simulink model "system_back_end"  (R2023a)
settings: Solver=VariableStepAuto  StartTime=0.0  StopTime=10.0  RelTol=1e-3
settings Model: Creator=Cinovasi  LastModifiedBy=Cinovasi

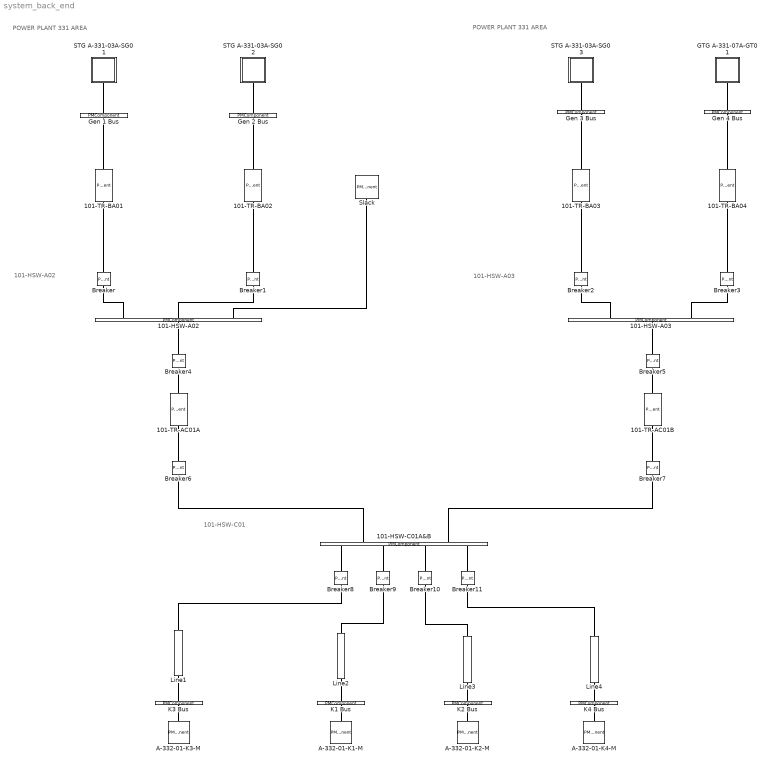
== system system_back_end ==
  note: 101-HSW-A03
  note: 101-HSW-A02
  note: 101-HSW-C01
  note: POWER PLANT 331 AREA
  note: POWER PLANT 331 AREA
  101-HSW-A02 : PMComponent  Tag=PSATblock  Description=Connection  PhysicalDomain=psatdomain  LeftPortType=p1  RightPortType=p1  LConnTagsString=__newl0|__newl1|__newl2  RConnTagsString=__newr0  mask(Bus){in=3, out=1, p2q=33, p3_4q=[1.00  0.00], p5q=1, p6q=1}
      mask prompts: in "Number of inputs:"; out "Number of outputs:"; p2q "Voltage Rating [kV]"; p3_4q "Voltage initial guess [p.u.  rad]"; p5q "Area number"; p6q "Region number"
      mask help: Bus block.
      mask init:
      | fm_inout
      mask Callback p5q: fm_block
      mask Display: plot([0 1 1 0 0],[0 0 1 1 0])
  101-HSW-A03 : PMComponent  Tag=PSATblock  Description=Connection  PhysicalDomain=psatdomain  LeftPortType=p1  RightPortType=p1  LConnTagsString=__newl0|__newl1  RConnTagsString=__newr0  mask(Bus){in=2, out=1, p2q=33, p3_4q=[1.00  0.00], p5q=1, p6q=1}
      mask prompts: in "Number of inputs:"; out "Number of outputs:"; p2q "Voltage Rating [kV]"; p3_4q "Voltage initial guess [p.u.  rad]"; p5q "Area number"; p6q "Region number"
      mask help: Bus block.
      mask init:
      | fm_inout
      mask Callback p5q: fm_block
      mask Display: plot([0 1 1 0 0],[0 0 1 1 0])
  101-HSW-C01A&B : PMComponent  Tag=PSATblock  Description=Connection  PhysicalDomain=psatdomain  LeftPortType=p1  RightPortType=p1  LConnTagsString=__newl0|__newl1  RConnTagsString=__newr0|__newr1|__newr2|__newr3  mask(Bus){in=2, out=4, p2q=5, p3_4q=[1.00  0.00], p5q=1, p6q=1}
      mask prompts: in "Number of inputs:"; out "Number of outputs:"; p2q "Voltage Rating [kV]"; p3_4q "Voltage initial guess [p.u.  rad]"; p5q "Area number"; p6q "Region number"
      mask help: Bus block.
      mask init:
      | fm_inout
      mask Callback p5q: fm_block
      mask Display: plot([0 1 1 0 0],[0 0 1 1 0])
  101-TR-AC01A : PMComponent  Tag=PSATblock  Description=Power Flow  PhysicalDomain=psatdomain  LeftPortType=p1  RightPortType=p1  LConnTagsString=__newl0  RConnTagsString=__newr0  mask(Line){p3_4_5q=[40 33 50], p7q=33/7, p8q=0.01, p9q=0.20, p13_14_15q=[0.0  0.0  0.0], p16q=on}
      mask prompts: p3_4_5q "Power, Voltage and Frequency Ratings [MVA, kV, Hz]"; p7q "Primary and secondary voltage ratio [kV/kV]"; p8q "Resistance [p.u.]"; p9q "Reactance [p.u.]"; p13_14_15q "Imax, Pmax and Smax [p.u., p.u., p.u.]"; p16q "Connected"
      mask help: This block defines a transformer.
      mask init:
      | [x,y] = fm_draw('circle');
      | [x1,y1] = fm_draw('1');
      | [x2,y2] = fm_draw('2');
      mask Callback p16q: fm_block
      mask Display:
      | plot(x,y,x+1.4,y,[-1 -1.3],[0 0],[2.4 2.7],[0 0])
      | color('green')
      | plot(-0.1+0.65*x1,0.65*y1)
      | plot(1.5+0.65*x2,0.65*y2)
  101-TR-AC01B : PMComponent  Tag=PSATblock  Description=Power Flow  PhysicalDomain=psatdomain  LeftPortType=p1  RightPortType=p1  LConnTagsString=__newl0  RConnTagsString=__newr0  mask(Line){p3_4_5q=[40 33 50], p7q=33/7, p8q=0.01, p9q=0.20, p13_14_15q=[0.0  0.0  0.0], p16q=on}
      mask prompts: p3_4_5q "Power, Voltage and Frequency Ratings [MVA, kV, Hz]"; p7q "Primary and secondary voltage ratio [kV/kV]"; p8q "Resistance [p.u.]"; p9q "Reactance [p.u.]"; p13_14_15q "Imax, Pmax and Smax [p.u., p.u., p.u.]"; p16q "Connected"
      mask help: This block defines a transformer.
      mask init:
      | [x,y] = fm_draw('circle');
      | [x1,y1] = fm_draw('1');
      | [x2,y2] = fm_draw('2');
      mask Callback p16q: fm_block
      mask Display:
      | plot(x,y,x+1.4,y,[-1 -1.3],[0 0],[2.4 2.7],[0 0])
      | color('green')
      | plot(-0.1+0.65*x1,0.65*y1)
      | plot(1.5+0.65*x2,0.65*y2)
  101-TR-BA01 : PMComponent  Tag=PSATblock  Description=Power Flow  PhysicalDomain=psatdomain  LeftPortType=p1  RightPortType=p1  LConnTagsString=__newl0  RConnTagsString=__newr0  mask(Line){p3_4_5q=[40 11 50], p7q=11/20, p8q=0.01, p9q=0.20, p13_14_15q=[0.0  0.0  0.0], p16q=on}
      mask prompts: p3_4_5q "Power, Voltage and Frequency Ratings [MVA, kV, Hz]"; p7q "Primary and secondary voltage ratio [kV/kV]"; p8q "Resistance [p.u.]"; p9q "Reactance [p.u.]"; p13_14_15q "Imax, Pmax and Smax [p.u., p.u., p.u.]"; p16q "Connected"
      mask help: This block defines a transformer.
      mask init:
      | [x,y] = fm_draw('circle');
      | [x1,y1] = fm_draw('1');
      | [x2,y2] = fm_draw('2');
      mask Callback p16q: fm_block
      mask Display:
      | plot(x,y,x+1.4,y,[-1 -1.3],[0 0],[2.4 2.7],[0 0])
      | color('green')
      | plot(-0.1+0.65*x1,0.65*y1)
      | plot(1.5+0.65*x2,0.65*y2)
  101-TR-BA02 : PMComponent  Tag=PSATblock  Description=Power Flow  PhysicalDomain=psatdomain  LeftPortType=p1  RightPortType=p1  LConnTagsString=__newl0  RConnTagsString=__newr0  mask(Line){p3_4_5q=[40 11 50], p7q=11/20, p8q=0.01, p9q=0.20, p13_14_15q=[0.0  0.0  0.0], p16q=on}
      mask prompts: p3_4_5q "Power, Voltage and Frequency Ratings [MVA, kV, Hz]"; p7q "Primary and secondary voltage ratio [kV/kV]"; p8q "Resistance [p.u.]"; p9q "Reactance [p.u.]"; p13_14_15q "Imax, Pmax and Smax [p.u., p.u., p.u.]"; p16q "Connected"
      mask help: This block defines a transformer.
      mask init:
      | [x,y] = fm_draw('circle');
      | [x1,y1] = fm_draw('1');
      | [x2,y2] = fm_draw('2');
      mask Callback p16q: fm_block
      mask Display:
      | plot(x,y,x+1.4,y,[-1 -1.3],[0 0],[2.4 2.7],[0 0])
      | color('green')
      | plot(-0.1+0.65*x1,0.65*y1)
      | plot(1.5+0.65*x2,0.65*y2)
  101-TR-BA03 : PMComponent  Tag=PSATblock  Description=Power Flow  PhysicalDomain=psatdomain  LeftPortType=p1  RightPortType=p1  LConnTagsString=__newl0  RConnTagsString=__newr0  mask(Line){p3_4_5q=[40 11 50], p7q=11/20, p8q=0.01, p9q=0.20, p13_14_15q=[0.0  0.0  0.0], p16q=on}
      mask prompts: p3_4_5q "Power, Voltage and Frequency Ratings [MVA, kV, Hz]"; p7q "Primary and secondary voltage ratio [kV/kV]"; p8q "Resistance [p.u.]"; p9q "Reactance [p.u.]"; p13_14_15q "Imax, Pmax and Smax [p.u., p.u., p.u.]"; p16q "Connected"
      mask help: This block defines a transformer.
      mask init:
      | [x,y] = fm_draw('circle');
      | [x1,y1] = fm_draw('1');
      | [x2,y2] = fm_draw('2');
      mask Callback p16q: fm_block
      mask Display:
      | plot(x,y,x+1.4,y,[-1 -1.3],[0 0],[2.4 2.7],[0 0])
      | color('green')
      | plot(-0.1+0.65*x1,0.65*y1)
      | plot(1.5+0.65*x2,0.65*y2)
  101-TR-BA04 : PMComponent  Tag=PSATblock  Description=Power Flow  PhysicalDomain=psatdomain  LeftPortType=p1  RightPortType=p1  LConnTagsString=__newl0  RConnTagsString=__newr0  mask(Line){p3_4_5q=[40 11 50], p7q=11/20, p8q=0.01, p9q=0.20, p13_14_15q=[0.0  0.0  0.0], p16q=on}
      mask prompts: p3_4_5q "Power, Voltage and Frequency Ratings [MVA, kV, Hz]"; p7q "Primary and secondary voltage ratio [kV/kV]"; p8q "Resistance [p.u.]"; p9q "Reactance [p.u.]"; p13_14_15q "Imax, Pmax and Smax [p.u., p.u., p.u.]"; p16q "Connected"
      mask help: This block defines a transformer.
      mask init:
      | [x,y] = fm_draw('circle');
      | [x1,y1] = fm_draw('1');
      | [x2,y2] = fm_draw('2');
      mask Callback p16q: fm_block
      mask Display:
      | plot(x,y,x+1.4,y,[-1 -1.3],[0 0],[2.4 2.7],[0 0])
      | color('green')
      | plot(-0.1+0.65*x1,0.65*y1)
      | plot(1.5+0.65*x2,0.65*y2)
  A-332-01-K1-M : PMComponent  Tag=PSATblock  Description=Machines  PhysicalDomain=psatdomain  LeftPortType=p1  RightPortType=p1  LConnTagsString=__newl0  mask(Ind){p2_3_4q=[40 6.6 50], p5q=3, p6q=off, p7q=0.01, p8q=0.15, p9_10q=[0.05  0.15], p11_12q=[0.001  0.04], p13q=5.00, p14q=3.00, p15_16_17q=[1.00  0.00  0.00], p18q=0, p19q=off, p20q=on}
      mask prompts: p2_3_4q "Power, Voltage and Frequency Ratings [MVA, kV, Hz]"; p5q "Dynamic Order"; p6q "Start up"; p7q "Stator Resistance Rs [p.u.]"; p8q "Stator Reactance Xs [p.u.]"; p9_10q "First Cage Resitance Rr1 and Reactance  Xr1 [p.u. p.u.]"; p11_12q "Second Cage Resistance Rr2 and Reactance Xr2 [p.u.  p.u.]"; p13q "Magnetization Reactance Xm [p.u.]"; p14q "Inertia Constant Hm [kWs/kVA]"; p15_16_17q "Mechanical Torque coefficients [a, b, c] [p.u.  p.u.  p.u.]"; p18q "Start up time"; p19q "Allow working as brake"; p20q "Connected"
      mask help:
      | This block defines an asynchronous machine.
      |
      | Order 1:  mechanical equation
      | Order 3:  single cage
      | Order 5:  double cage
      mask init:
      | [x,y] = fm_draw('circle');
      | [xs,ys] = fm_draw('sinus');
      mask TypeOptions p5q: 1 | 3 | 5
      mask Callback p5q: fm_block
      mask Callback p20q: fm_block
      mask Display:
      | plot(x+1.4,y,0.12*xs+1,0.15*ys-0.6)
      | color('blue')
      | plot([1 1 1.4 1.8 1.8],[-0.05 0.7 0.4 0.7 -0.05])
  A-332-01-K2-M : PMComponent  Tag=PSATblock  Description=Machines  PhysicalDomain=psatdomain  LeftPortType=p1  RightPortType=p1  LConnTagsString=__newl0  mask(Ind){p2_3_4q=[40 6.6 50], p5q=3, p6q=off, p7q=0.01, p8q=0.15, p9_10q=[0.05  0.15], p11_12q=[0.001  0.04], p13q=5.00, p14q=3.00, p15_16_17q=[1.00  0.00  0.00], p18q=0, p19q=off, p20q=on}
      mask prompts: p2_3_4q "Power, Voltage and Frequency Ratings [MVA, kV, Hz]"; p5q "Dynamic Order"; p6q "Start up"; p7q "Stator Resistance Rs [p.u.]"; p8q "Stator Reactance Xs [p.u.]"; p9_10q "First Cage Resitance Rr1 and Reactance  Xr1 [p.u. p.u.]"; p11_12q "Second Cage Resistance Rr2 and Reactance Xr2 [p.u.  p.u.]"; p13q "Magnetization Reactance Xm [p.u.]"; p14q "Inertia Constant Hm [kWs/kVA]"; p15_16_17q "Mechanical Torque coefficients [a, b, c] [p.u.  p.u.  p.u.]"; p18q "Start up time"; p19q "Allow working as brake"; p20q "Connected"
      mask help:
      | This block defines an asynchronous machine.
      |
      | Order 1:  mechanical equation
      | Order 3:  single cage
      | Order 5:  double cage
      mask init:
      | [x,y] = fm_draw('circle');
      | [xs,ys] = fm_draw('sinus');
      mask TypeOptions p5q: 1 | 3 | 5
      mask Callback p5q: fm_block
      mask Callback p20q: fm_block
      mask Display:
      | plot(x+1.4,y,0.12*xs+1,0.15*ys-0.6)
      | color('blue')
      | plot([1 1 1.4 1.8 1.8],[-0.05 0.7 0.4 0.7 -0.05])
  A-332-01-K3-M : PMComponent  Tag=PSATblock  Description=Machines  PhysicalDomain=psatdomain  LeftPortType=p1  RightPortType=p1  LConnTagsString=__newl0  mask(Ind){p2_3_4q=[40 6.6 50], p5q=3, p6q=off, p7q=0.01, p8q=0.15, p9_10q=[0.05  0.15], p11_12q=[0.001  0.04], p13q=5.00, p14q=3.00, p15_16_17q=[1.00  0.00  0.00], p18q=0, p19q=off, p20q=on}
      mask prompts: p2_3_4q "Power, Voltage and Frequency Ratings [MVA, kV, Hz]"; p5q "Dynamic Order"; p6q "Start up"; p7q "Stator Resistance Rs [p.u.]"; p8q "Stator Reactance Xs [p.u.]"; p9_10q "First Cage Resitance Rr1 and Reactance  Xr1 [p.u. p.u.]"; p11_12q "Second Cage Resistance Rr2 and Reactance Xr2 [p.u.  p.u.]"; p13q "Magnetization Reactance Xm [p.u.]"; p14q "Inertia Constant Hm [kWs/kVA]"; p15_16_17q "Mechanical Torque coefficients [a, b, c] [p.u.  p.u.  p.u.]"; p18q "Start up time"; p19q "Allow working as brake"; p20q "Connected"
      mask help:
      | This block defines an asynchronous machine.
      |
      | Order 1:  mechanical equation
      | Order 3:  single cage
      | Order 5:  double cage
      mask init:
      | [x,y] = fm_draw('circle');
      | [xs,ys] = fm_draw('sinus');
      mask TypeOptions p5q: 1 | 3 | 5
      mask Callback p5q: fm_block
      mask Callback p20q: fm_block
      mask Display:
      | plot(x+1.4,y,0.12*xs+1,0.15*ys-0.6)
      | color('blue')
      | plot([1 1 1.4 1.8 1.8],[-0.05 0.7 0.4 0.7 -0.05])
  A-332-01-K4-M : PMComponent  Tag=PSATblock  Description=Machines  PhysicalDomain=psatdomain  LeftPortType=p1  RightPortType=p1  LConnTagsString=__newl0  mask(Ind){p2_3_4q=[40 6.6 50], p5q=3, p6q=off, p7q=0.01, p8q=0.15, p9_10q=[0.05  0.15], p11_12q=[0.001  0.04], p13q=5.00, p14q=3.00, p15_16_17q=[1.00  0.00  0.00], p18q=0, p19q=off, p20q=on}
      mask prompts: p2_3_4q "Power, Voltage and Frequency Ratings [MVA, kV, Hz]"; p5q "Dynamic Order"; p6q "Start up"; p7q "Stator Resistance Rs [p.u.]"; p8q "Stator Reactance Xs [p.u.]"; p9_10q "First Cage Resitance Rr1 and Reactance  Xr1 [p.u. p.u.]"; p11_12q "Second Cage Resistance Rr2 and Reactance Xr2 [p.u.  p.u.]"; p13q "Magnetization Reactance Xm [p.u.]"; p14q "Inertia Constant Hm [kWs/kVA]"; p15_16_17q "Mechanical Torque coefficients [a, b, c] [p.u.  p.u.  p.u.]"; p18q "Start up time"; p19q "Allow working as brake"; p20q "Connected"
      mask help:
      | This block defines an asynchronous machine.
      |
      | Order 1:  mechanical equation
      | Order 3:  single cage
      | Order 5:  double cage
      mask init:
      | [x,y] = fm_draw('circle');
      | [xs,ys] = fm_draw('sinus');
      mask TypeOptions p5q: 1 | 3 | 5
      mask Callback p5q: fm_block
      mask Callback p20q: fm_block
      mask Display:
      | plot(x+1.4,y,0.12*xs+1,0.15*ys-0.6)
      | color('blue')
      | plot([1 1 1.4 1.8 1.8],[-0.05 0.7 0.4 0.7 -0.05])
  Breaker : PMComponent  Tag=PSATblock  Description=Faults & Breakers  PhysicalDomain=psatdomain  LeftPortType=p1  RightPortType=p1  LConnTagsString=__newl0  RConnTagsString=__newr0  mask(Breaker){p3_4_5q=[40 34.5  50], p6q=on, p7q=0.00, p8q=0.00, p9q=on, p10q=on}
      mask prompts: p3_4_5q "Power, Voltage and Frequency Ratings [MVA, kV, Hz]"; p6q "Initially close"; p7q "First intervention time [s]"; p8q "Second intervention time [s]"; p9q "Apply first intervention"; p10q "Apply second intervention"
      mask help: This block defines a transmission line breaker.
      mask Callback p6q: fm_block
      mask Display: plot([1 2 2 1 1],[-1 -1 1 1 -1]),color('red'),plot([1 2],[-1 1],[2 1],[-1 1])
  Breaker1 : PMComponent  Tag=PSATblock  Description=Faults & Breakers  PhysicalDomain=psatdomain  LeftPortType=p1  RightPortType=p1  LConnTagsString=__newl0  RConnTagsString=__newr0  mask(Breaker){p3_4_5q=[40 34.5  50], p6q=on, p7q=0.00, p8q=0.00, p9q=on, p10q=on}
      mask prompts: p3_4_5q "Power, Voltage and Frequency Ratings [MVA, kV, Hz]"; p6q "Initially close"; p7q "First intervention time [s]"; p8q "Second intervention time [s]"; p9q "Apply first intervention"; p10q "Apply second intervention"
      mask help: This block defines a transmission line breaker.
      mask Callback p6q: fm_block
      mask Display: plot([1 2 2 1 1],[-1 -1 1 1 -1]),color('red'),plot([1 2],[-1 1],[2 1],[-1 1])
  Breaker10 : PMComponent  Tag=PSATblock  Description=Faults & Breakers  PhysicalDomain=psatdomain  LeftPortType=p1  RightPortType=p1  LConnTagsString=__newl0  RConnTagsString=__newr0  mask(Breaker){p3_4_5q=[40 6.6  50], p6q=on, p7q=0.00, p8q=0.00, p9q=on, p10q=on}
      mask prompts: p3_4_5q "Power, Voltage and Frequency Ratings [MVA, kV, Hz]"; p6q "Initially close"; p7q "First intervention time [s]"; p8q "Second intervention time [s]"; p9q "Apply first intervention"; p10q "Apply second intervention"
      mask help: This block defines a transmission line breaker.
      mask Callback p6q: fm_block
      mask Display: plot([1 2 2 1 1],[-1 -1 1 1 -1]),color('red'),plot([1 2],[-1 1],[2 1],[-1 1])
  Breaker11 : PMComponent  Tag=PSATblock  Description=Faults & Breakers  PhysicalDomain=psatdomain  LeftPortType=p1  RightPortType=p1  LConnTagsString=__newl0  RConnTagsString=__newr0  mask(Breaker){p3_4_5q=[40 6.6  50], p6q=on, p7q=0.00, p8q=0.00, p9q=on, p10q=on}
      mask prompts: p3_4_5q "Power, Voltage and Frequency Ratings [MVA, kV, Hz]"; p6q "Initially close"; p7q "First intervention time [s]"; p8q "Second intervention time [s]"; p9q "Apply first intervention"; p10q "Apply second intervention"
      mask help: This block defines a transmission line breaker.
      mask Callback p6q: fm_block
      mask Display: plot([1 2 2 1 1],[-1 -1 1 1 -1]),color('red'),plot([1 2],[-1 1],[2 1],[-1 1])
  Breaker2 : PMComponent  Tag=PSATblock  Description=Faults & Breakers  PhysicalDomain=psatdomain  LeftPortType=p1  RightPortType=p1  LConnTagsString=__newl0  RConnTagsString=__newr0  mask(Breaker){p3_4_5q=[40 34.5  50], p6q=on, p7q=0.00, p8q=0.00, p9q=on, p10q=on}
      mask prompts: p3_4_5q "Power, Voltage and Frequency Ratings [MVA, kV, Hz]"; p6q "Initially close"; p7q "First intervention time [s]"; p8q "Second intervention time [s]"; p9q "Apply first intervention"; p10q "Apply second intervention"
      mask help: This block defines a transmission line breaker.
      mask Callback p6q: fm_block
      mask Display: plot([1 2 2 1 1],[-1 -1 1 1 -1]),color('red'),plot([1 2],[-1 1],[2 1],[-1 1])
  Breaker3 : PMComponent  Tag=PSATblock  Description=Faults & Breakers  PhysicalDomain=psatdomain  LeftPortType=p1  RightPortType=p1  LConnTagsString=__newl0  RConnTagsString=__newr0  mask(Breaker){p3_4_5q=[40 34.5  50], p6q=on, p7q=0.00, p8q=0.00, p9q=on, p10q=on}
      mask prompts: p3_4_5q "Power, Voltage and Frequency Ratings [MVA, kV, Hz]"; p6q "Initially close"; p7q "First intervention time [s]"; p8q "Second intervention time [s]"; p9q "Apply first intervention"; p10q "Apply second intervention"
      mask help: This block defines a transmission line breaker.
      mask Callback p6q: fm_block
      mask Display: plot([1 2 2 1 1],[-1 -1 1 1 -1]),color('red'),plot([1 2],[-1 1],[2 1],[-1 1])
  Breaker4 : PMComponent  Tag=PSATblock  Description=Faults & Breakers  PhysicalDomain=psatdomain  LeftPortType=p1  RightPortType=p1  LConnTagsString=__newl0  RConnTagsString=__newr0  mask(Breaker){p3_4_5q=[40 34.5  50], p6q=on, p7q=0.00, p8q=0.00, p9q=on, p10q=on}
      mask prompts: p3_4_5q "Power, Voltage and Frequency Ratings [MVA, kV, Hz]"; p6q "Initially close"; p7q "First intervention time [s]"; p8q "Second intervention time [s]"; p9q "Apply first intervention"; p10q "Apply second intervention"
      mask help: This block defines a transmission line breaker.
      mask Callback p6q: fm_block
      mask Display: plot([1 2 2 1 1],[-1 -1 1 1 -1]),color('red'),plot([1 2],[-1 1],[2 1],[-1 1])
  Breaker5 : PMComponent  Tag=PSATblock  Description=Faults & Breakers  PhysicalDomain=psatdomain  LeftPortType=p1  RightPortType=p1  LConnTagsString=__newl0  RConnTagsString=__newr0  mask(Breaker){p3_4_5q=[40 34.5  50], p6q=on, p7q=0.00, p8q=0.00, p9q=on, p10q=on}
      mask prompts: p3_4_5q "Power, Voltage and Frequency Ratings [MVA, kV, Hz]"; p6q "Initially close"; p7q "First intervention time [s]"; p8q "Second intervention time [s]"; p9q "Apply first intervention"; p10q "Apply second intervention"
      mask help: This block defines a transmission line breaker.
      mask Callback p6q: fm_block
      mask Display: plot([1 2 2 1 1],[-1 -1 1 1 -1]),color('red'),plot([1 2],[-1 1],[2 1],[-1 1])
  Breaker6 : PMComponent  Tag=PSATblock  Description=Faults & Breakers  PhysicalDomain=psatdomain  LeftPortType=p1  RightPortType=p1  LConnTagsString=__newl0  RConnTagsString=__newr0  mask(Breaker){p3_4_5q=[40 6.6  50], p6q=on, p7q=0.00, p8q=0.00, p9q=on, p10q=on}
      mask prompts: p3_4_5q "Power, Voltage and Frequency Ratings [MVA, kV, Hz]"; p6q "Initially close"; p7q "First intervention time [s]"; p8q "Second intervention time [s]"; p9q "Apply first intervention"; p10q "Apply second intervention"
      mask help: This block defines a transmission line breaker.
      mask Callback p6q: fm_block
      mask Display: plot([1 2 2 1 1],[-1 -1 1 1 -1]),color('red'),plot([1 2],[-1 1],[2 1],[-1 1])
  Breaker7 : PMComponent  Tag=PSATblock  Description=Faults & Breakers  PhysicalDomain=psatdomain  LeftPortType=p1  RightPortType=p1  LConnTagsString=__newl0  RConnTagsString=__newr0  mask(Breaker){p3_4_5q=[40 6.6  50], p6q=on, p7q=0.00, p8q=0.00, p9q=on, p10q=on}
      mask prompts: p3_4_5q "Power, Voltage and Frequency Ratings [MVA, kV, Hz]"; p6q "Initially close"; p7q "First intervention time [s]"; p8q "Second intervention time [s]"; p9q "Apply first intervention"; p10q "Apply second intervention"
      mask help: This block defines a transmission line breaker.
      mask Callback p6q: fm_block
      mask Display: plot([1 2 2 1 1],[-1 -1 1 1 -1]),color('red'),plot([1 2],[-1 1],[2 1],[-1 1])
  Breaker8 : PMComponent  Tag=PSATblock  Description=Faults & Breakers  PhysicalDomain=psatdomain  LeftPortType=p1  RightPortType=p1  LConnTagsString=__newl0  RConnTagsString=__newr0  mask(Breaker){p3_4_5q=[40 6.6  50], p6q=on, p7q=0.00, p8q=0.00, p9q=on, p10q=on}
      mask prompts: p3_4_5q "Power, Voltage and Frequency Ratings [MVA, kV, Hz]"; p6q "Initially close"; p7q "First intervention time [s]"; p8q "Second intervention time [s]"; p9q "Apply first intervention"; p10q "Apply second intervention"
      mask help: This block defines a transmission line breaker.
      mask Callback p6q: fm_block
      mask Display: plot([1 2 2 1 1],[-1 -1 1 1 -1]),color('red'),plot([1 2],[-1 1],[2 1],[-1 1])
  Breaker9 : PMComponent  Tag=PSATblock  Description=Faults & Breakers  PhysicalDomain=psatdomain  LeftPortType=p1  RightPortType=p1  LConnTagsString=__newl0  RConnTagsString=__newr0  mask(Breaker){p3_4_5q=[40 6.6  50], p6q=on, p7q=0.00, p8q=0.00, p9q=on, p10q=on}
      mask prompts: p3_4_5q "Power, Voltage and Frequency Ratings [MVA, kV, Hz]"; p6q "Initially close"; p7q "First intervention time [s]"; p8q "Second intervention time [s]"; p9q "Apply first intervention"; p10q "Apply second intervention"
      mask help: This block defines a transmission line breaker.
      mask Callback p6q: fm_block
      mask Display: plot([1 2 2 1 1],[-1 -1 1 1 -1]),color('red'),plot([1 2],[-1 1],[2 1],[-1 1])
  GTG A-331-07A-GT01 : Subsystem  Tag=PSATblock  Description=Machines  mask(Syn){p2_3_4q=[37.5 11 50], p5q=3, p7_6q=[0.001  0.05], p8_9_10q=[1.90  0.302  0.204], p11_12q=[8.00  0.04], p13_14_15q=[1.70  0.50  0.30], p16_17q=[0.80  0.02], p18_19q=[10.00  0.00], p20_21q=[0.00  0.00], p22_23q=[1.00  1.00], p24q=0.002, p25_26q=[0 0], in=0, p27q=1, p28q=on}
      mask prompts: p2_3_4q "Power, voltage and frequency ratings [MVA, kV, Hz]"; p5q "Machine Dynamic Order"; p7_6q "resistance ra and leakage reactance xl [p.u. p.u.]"; p8_9_10q "d-axis reactances Xd, X'd X"d [p.u.,p.u.,p.u.]"; p11_12q "d-axis open circuit time constants T'd0 and T"d0 [s, s]"; p13_14_15q "q-axis reactances Xq, X'q, X"q [p.u.  p.u.  p.u.]"; p16_17q "q-axis open circuit time constants T'q0 and T"q0 [s s]"; p18_19q "Inertia (M = 2H) and Damping [s, p.u.]"; p20_21q "Speed and active power additional signals Kw and Kp [p.u., p.u.]"; p22_23q "Percentage of active and reactive powers at bus [p.u. p.u.]"; p24q "d-axis additional circuit leakage time constant Taa [s]"; p25_26q "Saturation coefficients S(1.0) and S(1.2)"; in "Number of input signals"; p27q "COI number"; p28q "Connected"
      mask help: This block defines a fourth order synchronous machine.
      mask init:
      | fm_inout
      | [x,y] = fm_draw('circle');
      | [xg,yg] = fm_draw('G');
      | [xs,ys] = fm_draw('sinus');
      mask TypeOptions p5q: 8 | 6 | 5.3 | 5.2 | 5.1 | 4 | 3 | 2
      mask Callback p5q: fm_block
      mask TypeOptions in: 0 | 1 | 2
      mask Callback p28q: fm_block
      mask Display:
      | plot(x+1.4,y,0.12*xs+1,0.15*ys-0.6)
      | color('blue')
      | plot(1.4+0.45*xg,0.3+0.45*yg)
  Gen 1 Bus : PMComponent  Tag=PSATblock  Description=Connection  PhysicalDomain=psatdomain  LeftPortType=p1  RightPortType=p1  LConnTagsString=__newl0  RConnTagsString=__newr0  mask(Bus){in=1, out=1, p2q=12, p3_4q=[1.00  0.00], p5q=1, p6q=1}
      mask prompts: in "Number of inputs:"; out "Number of outputs:"; p2q "Voltage Rating [kV]"; p3_4q "Voltage initial guess [p.u.  rad]"; p5q "Area number"; p6q "Region number"
      mask help: Bus block.
      mask init:
      | fm_inout
      mask Callback p5q: fm_block
      mask Display: plot([0 1 1 0 0],[0 0 1 1 0])
  Gen 2 Bus : PMComponent  Tag=PSATblock  Description=Connection  PhysicalDomain=psatdomain  LeftPortType=p1  RightPortType=p1  LConnTagsString=__newl0  RConnTagsString=__newr0  mask(Bus){in=1, out=1, p2q=13, p3_4q=[1.00  0.00], p5q=1, p6q=1}
      mask prompts: in "Number of inputs:"; out "Number of outputs:"; p2q "Voltage Rating [kV]"; p3_4q "Voltage initial guess [p.u.  rad]"; p5q "Area number"; p6q "Region number"
      mask help: Bus block.
      mask init:
      | fm_inout
      mask Callback p5q: fm_block
      mask Display: plot([0 1 1 0 0],[0 0 1 1 0])
  Gen 3 Bus : PMComponent  Tag=PSATblock  Description=Connection  PhysicalDomain=psatdomain  LeftPortType=p1  RightPortType=p1  LConnTagsString=__newl0  RConnTagsString=__newr0  mask(Bus){in=1, out=1, p2q=14, p3_4q=[1.00  0.00], p5q=1, p6q=1}
      mask prompts: in "Number of inputs:"; out "Number of outputs:"; p2q "Voltage Rating [kV]"; p3_4q "Voltage initial guess [p.u.  rad]"; p5q "Area number"; p6q "Region number"
      mask help: Bus block.
      mask init:
      | fm_inout
      mask Callback p5q: fm_block
      mask Display: plot([0 1 1 0 0],[0 0 1 1 0])
  Gen 4 Bus : PMComponent  Tag=PSATblock  Description=Connection  PhysicalDomain=psatdomain  LeftPortType=p1  RightPortType=p1  LConnTagsString=__newl0  RConnTagsString=__newr0  mask(Bus){in=1, out=1, p2q=15, p3_4q=[1.00  0.00], p5q=1, p6q=1}
      mask prompts: in "Number of inputs:"; out "Number of outputs:"; p2q "Voltage Rating [kV]"; p3_4q "Voltage initial guess [p.u.  rad]"; p5q "Area number"; p6q "Region number"
      mask help: Bus block.
      mask init:
      | fm_inout
      mask Callback p5q: fm_block
      mask Display: plot([0 1 1 0 0],[0 0 1 1 0])
  K1 Bus : PMComponent  Tag=PSATblock  Description=Connection  PhysicalDomain=psatdomain  LeftPortType=p1  RightPortType=p1  LConnTagsString=__newl0  RConnTagsString=__newr0  mask(Bus){in=1, out=1, p2q=6.6, p3_4q=[1.00  0.00], p5q=1, p6q=1}
      mask prompts: in "Number of inputs:"; out "Number of outputs:"; p2q "Voltage Rating [kV]"; p3_4q "Voltage initial guess [p.u.  rad]"; p5q "Area number"; p6q "Region number"
      mask help: Bus block.
      mask init:
      | fm_inout
      mask Callback p5q: fm_block
      mask Display: plot([0 1 1 0 0],[0 0 1 1 0])
  K2 Bus : PMComponent  Tag=PSATblock  Description=Connection  PhysicalDomain=psatdomain  LeftPortType=p1  RightPortType=p1  LConnTagsString=__newl0  RConnTagsString=__newr0  mask(Bus){in=1, out=1, p2q=6.6, p3_4q=[1.00  0.00], p5q=1, p6q=1}
      mask prompts: in "Number of inputs:"; out "Number of outputs:"; p2q "Voltage Rating [kV]"; p3_4q "Voltage initial guess [p.u.  rad]"; p5q "Area number"; p6q "Region number"
      mask help: Bus block.
      mask init:
      | fm_inout
      mask Callback p5q: fm_block
      mask Display: plot([0 1 1 0 0],[0 0 1 1 0])
  K3 Bus : PMComponent  Tag=PSATblock  Description=Connection  PhysicalDomain=psatdomain  LeftPortType=p1  RightPortType=p1  LConnTagsString=__newl0  RConnTagsString=__newr0  mask(Bus){in=1, out=1, p2q=6.6, p3_4q=[1.00  0.00], p5q=1, p6q=1}
      mask prompts: in "Number of inputs:"; out "Number of outputs:"; p2q "Voltage Rating [kV]"; p3_4q "Voltage initial guess [p.u.  rad]"; p5q "Area number"; p6q "Region number"
      mask help: Bus block.
      mask init:
      | fm_inout
      mask Callback p5q: fm_block
      mask Display: plot([0 1 1 0 0],[0 0 1 1 0])
  K4 Bus : PMComponent  Tag=PSATblock  Description=Connection  PhysicalDomain=psatdomain  LeftPortType=p1  RightPortType=p1  LConnTagsString=__newl0  RConnTagsString=__newr0  mask(Bus){in=1, out=1, p2q=6.6, p3_4q=[1.00  0.00], p5q=1, p6q=1}
      mask prompts: in "Number of inputs:"; out "Number of outputs:"; p2q "Voltage Rating [kV]"; p3_4q "Voltage initial guess [p.u.  rad]"; p5q "Area number"; p6q "Region number"
      mask help: Bus block.
      mask init:
      | fm_inout
      mask Callback p5q: fm_block
      mask Display: plot([0 1 1 0 0],[0 0 1 1 0])
  Line1 : PMComponent  Tag=PSATblock  Description=Power Flow  PhysicalDomain=psatdomain  LeftPortType=p1  RightPortType=p1  LConnTagsString=__newl0  RConnTagsString=__newr0  mask(Line){p3_4_5q=[40  6.6  50], p6q=0, p8q=0.01, p9q=0.10, p10q=1e-3, p13_14_15q=[0.0  0.0  0.0], p16q=on}
      mask prompts: p3_4_5q "Power, Voltage and Frequency Ratings [MVA, kV, Hz]"; p6q "Length of line [km] (0 for p.u. parameters)"; p8q "Resistance [p.u. (Ohms/km)]"; p9q "Reactance [p.u. (H/km)]"; p10q "Susceptance [p.u. (F/km)]"; p13_14_15q "Imax, Pmax and Smax [p.u., p.u., p.u.]"; p16q "Connected"
      mask help: This block defines a pi model for a tree phase cable.
      mask init:
      | [x,y] = fm_draw('circle');
      | [x1,y1] = fm_draw('semicircle');
      mask Callback p16q: fm_block
      mask Display:
      | color('yellow')
      | plot(10+0.433*x,0.5+0.433*y)
      | plot(9.567+0.433*x,-0.25+0.433*y)
      | plot(10.433+0.433*x,-0.25+0.433*y)
      | color('black')
      | plot(-x1,y1)
      | plot(10+x,y,[0 10],[1 1],[0 10],[-1 -1])
  Line2 : PMComponent  Tag=PSATblock  Description=Power Flow  PhysicalDomain=psatdomain  LeftPortType=p1  RightPortType=p1  LConnTagsString=__newl0  RConnTagsString=__newr0  mask(Line){p3_4_5q=[40  6.6  50], p6q=0, p8q=0.01, p9q=0.10, p10q=1e-3, p13_14_15q=[0.0  0.0  0.0], p16q=on}
      mask prompts: p3_4_5q "Power, Voltage and Frequency Ratings [MVA, kV, Hz]"; p6q "Length of line [km] (0 for p.u. parameters)"; p8q "Resistance [p.u. (Ohms/km)]"; p9q "Reactance [p.u. (H/km)]"; p10q "Susceptance [p.u. (F/km)]"; p13_14_15q "Imax, Pmax and Smax [p.u., p.u., p.u.]"; p16q "Connected"
      mask help: This block defines a pi model for a tree phase cable.
      mask init:
      | [x,y] = fm_draw('circle');
      | [x1,y1] = fm_draw('semicircle');
      mask Callback p16q: fm_block
      mask Display:
      | color('yellow')
      | plot(10+0.433*x,0.5+0.433*y)
      | plot(9.567+0.433*x,-0.25+0.433*y)
      | plot(10.433+0.433*x,-0.25+0.433*y)
      | color('black')
      | plot(-x1,y1)
      | plot(10+x,y,[0 10],[1 1],[0 10],[-1 -1])
  Line3 : PMComponent  Tag=PSATblock  Description=Power Flow  PhysicalDomain=psatdomain  LeftPortType=p1  RightPortType=p1  LConnTagsString=__newl0  RConnTagsString=__newr0  mask(Line){p3_4_5q=[40  6.6  50], p6q=0, p8q=0.01, p9q=0.10, p10q=1e-3, p13_14_15q=[0.0  0.0  0.0], p16q=on}
      mask prompts: p3_4_5q "Power, Voltage and Frequency Ratings [MVA, kV, Hz]"; p6q "Length of line [km] (0 for p.u. parameters)"; p8q "Resistance [p.u. (Ohms/km)]"; p9q "Reactance [p.u. (H/km)]"; p10q "Susceptance [p.u. (F/km)]"; p13_14_15q "Imax, Pmax and Smax [p.u., p.u., p.u.]"; p16q "Connected"
      mask help: This block defines a pi model for a tree phase cable.
      mask init:
      | [x,y] = fm_draw('circle');
      | [x1,y1] = fm_draw('semicircle');
      mask Callback p16q: fm_block
      mask Display:
      | color('yellow')
      | plot(10+0.433*x,0.5+0.433*y)
      | plot(9.567+0.433*x,-0.25+0.433*y)
      | plot(10.433+0.433*x,-0.25+0.433*y)
      | color('black')
      | plot(-x1,y1)
      | plot(10+x,y,[0 10],[1 1],[0 10],[-1 -1])
  Line4 : PMComponent  Tag=PSATblock  Description=Power Flow  PhysicalDomain=psatdomain  LeftPortType=p1  RightPortType=p1  LConnTagsString=__newl0  RConnTagsString=__newr0  mask(Line){p3_4_5q=[40  6.6  50], p6q=0, p8q=0.01, p9q=0.10, p10q=1e-3, p13_14_15q=[0.0  0.0  0.0], p16q=on}
      mask prompts: p3_4_5q "Power, Voltage and Frequency Ratings [MVA, kV, Hz]"; p6q "Length of line [km] (0 for p.u. parameters)"; p8q "Resistance [p.u. (Ohms/km)]"; p9q "Reactance [p.u. (H/km)]"; p10q "Susceptance [p.u. (F/km)]"; p13_14_15q "Imax, Pmax and Smax [p.u., p.u., p.u.]"; p16q "Connected"
      mask help: This block defines a pi model for a tree phase cable.
      mask init:
      | [x,y] = fm_draw('circle');
      | [x1,y1] = fm_draw('semicircle');
      mask Callback p16q: fm_block
      mask Display:
      | color('yellow')
      | plot(10+0.433*x,0.5+0.433*y)
      | plot(9.567+0.433*x,-0.25+0.433*y)
      | plot(10.433+0.433*x,-0.25+0.433*y)
      | color('black')
      | plot(-x1,y1)
      | plot(10+x,y,[0 10],[1 1],[0 10],[-1 -1])
  STG A-331-03A-SG01 : Subsystem  Tag=PSATblock  Description=Machines  mask(Syn){p2_3_4q=[37.5 11 50], p5q=3, p7_6q=[0.001  0.05], p8_9_10q=[1.90  0.302  0.204], p11_12q=[8.00  0.04], p13_14_15q=[1.70  0.50  0.30], p16_17q=[0.80  0.02], p18_19q=[10.00  0.00], p20_21q=[0.00  0.00], p22_23q=[1.00  1.00], p24q=0.002, p25_26q=[0 0], in=0, p27q=1, p28q=on}
      mask prompts: p2_3_4q "Power, voltage and frequency ratings [MVA, kV, Hz]"; p5q "Machine Dynamic Order"; p7_6q "resistance ra and leakage reactance xl [p.u. p.u.]"; p8_9_10q "d-axis reactances Xd, X'd X"d [p.u.,p.u.,p.u.]"; p11_12q "d-axis open circuit time constants T'd0 and T"d0 [s, s]"; p13_14_15q "q-axis reactances Xq, X'q, X"q [p.u.  p.u.  p.u.]"; p16_17q "q-axis open circuit time constants T'q0 and T"q0 [s s]"; p18_19q "Inertia (M = 2H) and Damping [s, p.u.]"; p20_21q "Speed and active power additional signals Kw and Kp [p.u., p.u.]"; p22_23q "Percentage of active and reactive powers at bus [p.u. p.u.]"; p24q "d-axis additional circuit leakage time constant Taa [s]"; p25_26q "Saturation coefficients S(1.0) and S(1.2)"; in "Number of input signals"; p27q "COI number"; p28q "Connected"
      mask help: This block defines a fourth order synchronous machine.
      mask init:
      | fm_inout
      | [x,y] = fm_draw('circle');
      | [xg,yg] = fm_draw('G');
      | [xs,ys] = fm_draw('sinus');
      mask TypeOptions p5q: 8 | 6 | 5.3 | 5.2 | 5.1 | 4 | 3 | 2
      mask Callback p5q: fm_block
      mask TypeOptions in: 0 | 1 | 2
      mask Callback p28q: fm_block
      mask Display:
      | plot(x+1.4,y,0.12*xs+1,0.15*ys-0.6)
      | color('blue')
      | plot(1.4+0.45*xg,0.3+0.45*yg)
  STG A-331-03A-SG02 : Subsystem  Tag=PSATblock  Description=Machines  mask(Syn){p2_3_4q=[37.5 11 50], p5q=3, p7_6q=[0.001  0.05], p8_9_10q=[1.90  0.302  0.204], p11_12q=[8.00  0.04], p13_14_15q=[1.70  0.50  0.30], p16_17q=[0.80  0.02], p18_19q=[10.00  0.00], p20_21q=[0.00  0.00], p22_23q=[1.00  1.00], p24q=0.002, p25_26q=[0 0], in=0, p27q=1, p28q=on}
      mask prompts: p2_3_4q "Power, voltage and frequency ratings [MVA, kV, Hz]"; p5q "Machine Dynamic Order"; p7_6q "resistance ra and leakage reactance xl [p.u. p.u.]"; p8_9_10q "d-axis reactances Xd, X'd X"d [p.u.,p.u.,p.u.]"; p11_12q "d-axis open circuit time constants T'd0 and T"d0 [s, s]"; p13_14_15q "q-axis reactances Xq, X'q, X"q [p.u.  p.u.  p.u.]"; p16_17q "q-axis open circuit time constants T'q0 and T"q0 [s s]"; p18_19q "Inertia (M = 2H) and Damping [s, p.u.]"; p20_21q "Speed and active power additional signals Kw and Kp [p.u., p.u.]"; p22_23q "Percentage of active and reactive powers at bus [p.u. p.u.]"; p24q "d-axis additional circuit leakage time constant Taa [s]"; p25_26q "Saturation coefficients S(1.0) and S(1.2)"; in "Number of input signals"; p27q "COI number"; p28q "Connected"
      mask help: This block defines a fourth order synchronous machine.
      mask init:
      | fm_inout
      | [x,y] = fm_draw('circle');
      | [xg,yg] = fm_draw('G');
      | [xs,ys] = fm_draw('sinus');
      mask TypeOptions p5q: 8 | 6 | 5.3 | 5.2 | 5.1 | 4 | 3 | 2
      mask Callback p5q: fm_block
      mask TypeOptions in: 0 | 1 | 2
      mask Callback p28q: fm_block
      mask Display:
      | plot(x+1.4,y,0.12*xs+1,0.15*ys-0.6)
      | color('blue')
      | plot(1.4+0.45*xg,0.3+0.45*yg)
  STG A-331-03A-SG03 : Subsystem  Tag=PSATblock  Description=Machines  mask(Syn){p2_3_4q=[37.5 11 50], p5q=3, p7_6q=[0.001  0.05], p8_9_10q=[1.90  0.302  0.204], p11_12q=[8.00  0.04], p13_14_15q=[1.70  0.50  0.30], p16_17q=[0.80  0.02], p18_19q=[10.00  0.00], p20_21q=[0.00  0.00], p22_23q=[1.00  1.00], p24q=0.002, p25_26q=[0 0], in=0, p27q=1, p28q=on}
      mask prompts: p2_3_4q "Power, voltage and frequency ratings [MVA, kV, Hz]"; p5q "Machine Dynamic Order"; p7_6q "resistance ra and leakage reactance xl [p.u. p.u.]"; p8_9_10q "d-axis reactances Xd, X'd X"d [p.u.,p.u.,p.u.]"; p11_12q "d-axis open circuit time constants T'd0 and T"d0 [s, s]"; p13_14_15q "q-axis reactances Xq, X'q, X"q [p.u.  p.u.  p.u.]"; p16_17q "q-axis open circuit time constants T'q0 and T"q0 [s s]"; p18_19q "Inertia (M = 2H) and Damping [s, p.u.]"; p20_21q "Speed and active power additional signals Kw and Kp [p.u., p.u.]"; p22_23q "Percentage of active and reactive powers at bus [p.u. p.u.]"; p24q "d-axis additional circuit leakage time constant Taa [s]"; p25_26q "Saturation coefficients S(1.0) and S(1.2)"; in "Number of input signals"; p27q "COI number"; p28q "Connected"
      mask help: This block defines a fourth order synchronous machine.
      mask init:
      | fm_inout
      | [x,y] = fm_draw('circle');
      | [xg,yg] = fm_draw('G');
      | [xs,ys] = fm_draw('sinus');
      mask TypeOptions p5q: 8 | 6 | 5.3 | 5.2 | 5.1 | 4 | 3 | 2
      mask Callback p5q: fm_block
      mask TypeOptions in: 0 | 1 | 2
      mask Callback p28q: fm_block
      mask Display:
      | plot(x+1.4,y,0.12*xs+1,0.15*ys-0.6)
      | color('blue')
      | plot(1.4+0.45*xg,0.3+0.45*yg)
  Slack : PMComponent  Tag=PSATblock  Description=Power Flow  PhysicalDomain=psatdomain  LeftPortType=p1  RightPortType=p1  RConnTagsString=__newr0  mask(SW){p2_3q=[40  33], p4q=1.00, p5q=0.00, p6_7q=[1.5  -1.5], p8_9q=[1.1  0.9], p10q=0.80, p11q=1, p12q=on, p13q=on}
      mask prompts: p2_3q "Power and Voltage Ratings [MVA, kV]"; p4q "Voltage Magnitude [p.u.]"; p5q "Reference Phase Angle [rad]"; p6_7q "Qmax and Qmin [p.u.  p.u.]"; p8_9q "Vmax and Vmin  [p.u.  p.u.]"; p10q "Active Power Guess [p.u.]"; p11q "Loss Participation Factor"; p12q "Reference bus"; p13q "Connected"
      mask help:
      | This block defines a V-theta bus:
      |
      | V = V_des
      | theta = theta_des
      mask init:
      | [x,y] = fm_draw('circle');
      | [xt,yt] = fm_draw('theta');
      mask Callback p12q: fm_block
      mask Callback p13q: fm_block
      mask Display: plot([0 1 1 0 0],[0 0 1 1 0]), color('blue'), plot([0 1],[0 1],[0 1],[1 0],[0.5 1 0.5 0 0.5],[0 0.5 1 0.5 0])
  connections:
  Breaker/RConn1 -- 101-HSW-A02/LConn1
  Breaker1/RConn1 -- 101-HSW-A02/LConn2
  101-TR-BA02/LConn1 -- Gen 2 Bus/RConn1
  101-TR-BA01/RConn1 -- Breaker/LConn1
  101-TR-BA02/RConn1 -- Breaker1/LConn1
  101-TR-BA03/LConn1 -- Gen 3 Bus/RConn1
  101-TR-BA04/LConn1 -- Gen 4 Bus/RConn1
  101-TR-BA03/RConn1 -- Breaker2/LConn1
  101-TR-BA04/RConn1 -- Breaker3/LConn1
  Breaker2/RConn1 -- 101-HSW-A03/LConn1
  Breaker3/RConn1 -- 101-HSW-A03/LConn2
  101-HSW-A02/RConn1 -- Breaker4/LConn1
  Breaker4/RConn1 -- 101-TR-AC01A/LConn1
  101-HSW-A03/RConn1 -- Breaker5/LConn1
  101-TR-AC01B/LConn1 -- Breaker5/RConn1
  101-TR-AC01A/RConn1 -- Breaker6/LConn1
  101-TR-AC01B/RConn1 -- Breaker7/LConn1
  101-HSW-C01A&B/LConn1 -- Breaker6/RConn1
  101-HSW-C01A&B/LConn2 -- Breaker7/RConn1
  Breaker8/LConn1 -- 101-HSW-C01A&B/RConn1
  Breaker9/LConn1 -- 101-HSW-C01A&B/RConn2
  Breaker10/LConn1 -- 101-HSW-C01A&B/RConn3
  Breaker11/LConn1 -- 101-HSW-C01A&B/RConn4
  K1 Bus/LConn1 -- Line2/RConn1
  K2 Bus/RConn1 -- A-332-01-K2-M/LConn1
  K4 Bus/RConn1 -- A-332-01-K4-M/LConn1
  Slack/RConn1 -- 101-HSW-A02/LConn3
  Gen 1 Bus/RConn1 -- 101-TR-BA01/LConn1
  A-332-01-K3-M/LConn1 -- K3 Bus/RConn1
  Line1/LConn1 -- Breaker8/RConn1
  A-332-01-K1-M/LConn1 -- K1 Bus/RConn1
  Breaker10/RConn1 -- Line3/LConn1
  Line4/RConn1 -- K4 Bus/LConn1
  K3 Bus/LConn1 -- Line1/RConn1
  Line2/LConn1 -- Breaker9/RConn1
  Line3/RConn1 -- K2 Bus/LConn1
  Breaker11/RConn1 -- Line4/LConn1
  STG A-331-03A-SG01/RConn1 -- Gen 1 Bus/LConn1
  STG A-331-03A-SG02/RConn1 -- Gen 2 Bus/LConn1
  STG A-331-03A-SG03/RConn1 -- Gen 3 Bus/LConn1
  GTG A-331-07A-GT01/RConn1 -- Gen 4 Bus/LConn1

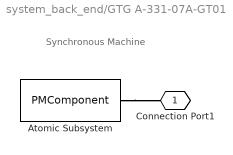
== system system_back_end/GTG A-331-07A-GT01 ==
  note: Synchronous Machine
  Atomic Subsystem : PMComponent  PhysicalDomain=psatdomain  LeftPortType=p1  RightPortType=p1  RConnTagsString=__newr0
  Connection Port1 : PMIOPort  Tag=PMCPort  Side=Right
  connections:
  Atomic Subsystem/RConn1 -- Connection Port1/RConn1

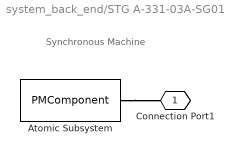
== system system_back_end/STG A-331-03A-SG01 ==
  note: Synchronous Machine
  Atomic Subsystem : PMComponent  PhysicalDomain=psatdomain  LeftPortType=p1  RightPortType=p1  RConnTagsString=__newr0
  Connection Port1 : PMIOPort  Tag=PMCPort  Side=Right
  connections:
  Atomic Subsystem/RConn1 -- Connection Port1/RConn1

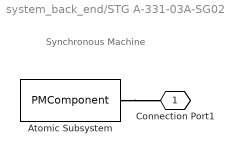
== system system_back_end/STG A-331-03A-SG02 ==
  note: Synchronous Machine
  Atomic Subsystem : PMComponent  PhysicalDomain=psatdomain  LeftPortType=p1  RightPortType=p1  RConnTagsString=__newr0
  Connection Port1 : PMIOPort  Tag=PMCPort  Side=Right
  connections:
  Atomic Subsystem/RConn1 -- Connection Port1/RConn1

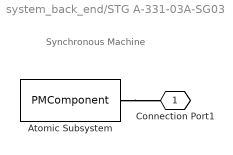
== system system_back_end/STG A-331-03A-SG03 ==
  note: Synchronous Machine
  Atomic Subsystem : PMComponent  PhysicalDomain=psatdomain  LeftPortType=p1  RightPortType=p1  RConnTagsString=__newr0
  Connection Port1 : PMIOPort  Tag=PMCPort  Side=Right
  connections:
  Atomic Subsystem/RConn1 -- Connection Port1/RConn1
